simulink model "sldemo_msfcn_frame"  (Simulink 7.6)
settings: Solver=FixedStepDiscrete  SolverMode=SingleTasking  StartTime=0.0  StopTime=20  FixedStep=1  RelTol=1e-3
settings Model: Creator=The MathWorks Inc.  ExtModeAutoUpdateStatusClock=off
settings DataIOCC: LimitDataPoints=off  SaveFormat=Structure  SignalLoggingName=logsOut
settings OptimizationCC: InitFltsAndDblsToZero=on  EfficientMapNaN2IntZero=off
settings DebuggingCC: SaveWithParameterizedLinksMsg=none  SignalResolutionControl=TryResolveAllWithWarning  SolverPrmCheckMsg=none  MultiTaskDSMMsg=warning  MultiTaskCondExecSysMsg=none
settings HardwareCC: TargetEndianess=LittleEndian  TargetHWDeviceType=MATLAB Host  ProdEqTarget=off
settings RTWCC: IncludeERTFirstTime=on
settings GRTTargetCC: TargetFcnLib=iso_c_tmw.mat

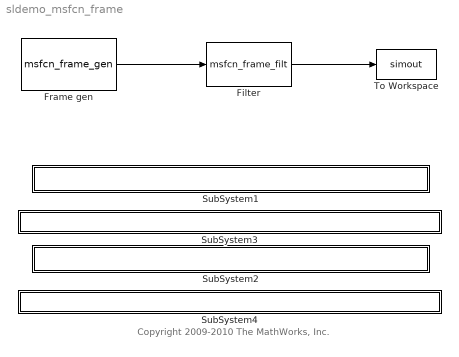
== system sldemo_msfcn_frame ==
  note: Copyright 2009-2010 The MathWorks, Inc.
  Filter : M-S-Function  FunctionName=msfcn_frame_filt  Parameters=t1,t2  mask(2-tap FIR filter){t1=0.5, t2=0.5}
      mask prompts: t1 "Tap1"; t2 "Tap2"
      mask help: Implements a two-tap FIR filter that can process both frame-based and sample-based signals.
      mask Display: disp('Simple filter')
  Frame gen : M-S-Function  FunctionName=msfcn_frame_gen  Parameters=Amplitude,nSample,Period,sampleTime  mask{Amplitude=[1 2 3 4], Period=4, nSample=8, sampleTime=1}
      mask prompts: Period "Period (samples)"; nSample "Samples per frame"; sampleTime "Sample time"
      mask help:
      | Generate frame-based square signals.
      | Specify the amplitude and the period of the signal. The duty cycle is fixed at 50%, less if the period is an odd number.
      | Then specify the number of samples in a frame (NS) and the sample time (TS) to obtain the frame rate as fr=1/(TS*NS).
      mask Display: disp('Square function\n(frame based)')
  SubSystem1 : Subsystem  mask{filename=msfcn_frame_filt.m}
      mask init:
      | x=sfundemo_maskdisp;
      settings: AttributesFormatString=\n  OpenFcn=sfundemo_openfcn
      mask Display: disp(x);
  SubSystem2 : Subsystem  mask{filename=msfcn_frame_gen.m}
      mask init:
      | x=sfundemo_maskdisp;
      settings: AttributesFormatString=\n  OpenFcn=sfundemo_openfcn
      mask Display: disp(x);
  SubSystem3 : Subsystem  mask{filename=msfcn_frame_filt.tlc}
      mask init:
      | x=sfundemo_maskdisp;
      settings: AttributesFormatString=\n  OpenFcn=sfundemo_openfcn
      mask Display: disp(x);
  SubSystem4 : Subsystem  mask{filename=msfcn_frame_gen.tlc}
      mask init:
      | x=sfundemo_maskdisp;
      settings: AttributesFormatString=\n  OpenFcn=sfundemo_openfcn
      mask Display: disp(x);
  To Workspace : ToWorkspace  VariableName=simout  SampleTime=-1  SaveFormat=Structure
  wires:
  Filter/1 -> To Workspace/1
  Frame gen/1 -> Filter/1

== system sldemo_msfcn_frame/SubSystem1 ==

== system sldemo_msfcn_frame/SubSystem2 ==

== system sldemo_msfcn_frame/SubSystem3 ==

== system sldemo_msfcn_frame/SubSystem4 ==
